simulink model "control_core"  (R2022b)
settings: Solver=FixedStepAuto  StartTime=0.0  StopTime=60  FixedStep=.01  RelTol=1e-3
undefined symbols (not defined in the file): airframe, CdProp, Cdx, Cdy, Cdz, Ct, Earth, g, Ixx, Iyy, Izz, Jr, larm, mass, WGS84
libraries: slpidlib x6, aerolibutil x3, vrlib x3, sharedtransform x2, shared6dof x2, simulink_extras x2, simulink x2, aerolibfltsims x1, aerolibtransform2 x1
(part 2 of 2)

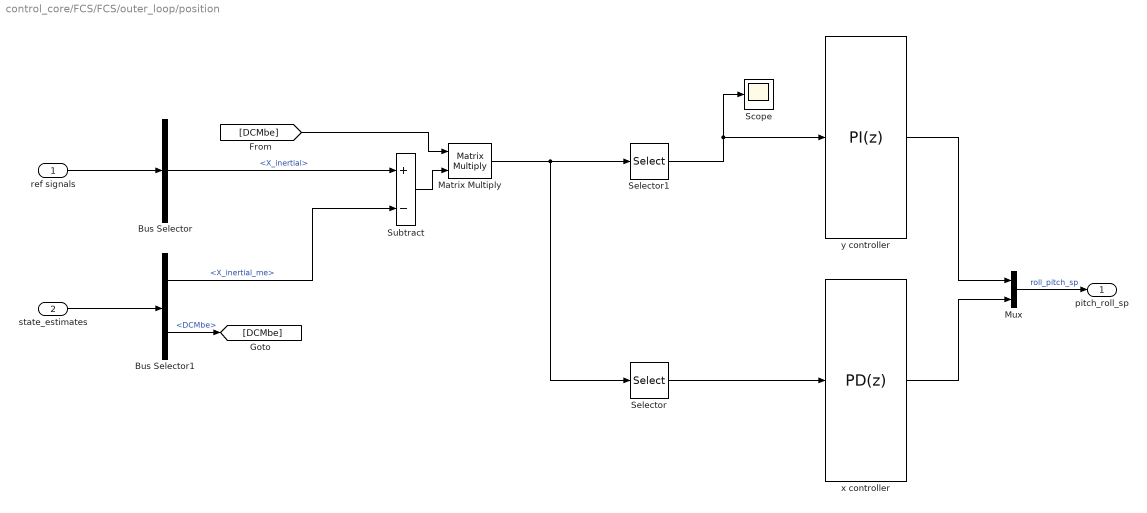
== system control_core/FCS/FCS/outer_loop/position ==
  ref signals : Inport
  state_estimates : Inport  Port=2
  Bus Selector : BusSelector  OutputSignals=X_inertial
  Bus Selector1 : BusSelector  OutputSignals=X_inertial_me,DCMbe
  Matrix Multiply : Product  Multiplication=Matrix(*)
  Mux : Mux  Inputs=2
  Scope : Scope
  Selector : Selector  InputPortWidth=3  IndexOptions=Index vector (dialog)  Indices=[1]  OutputSizes=1
  Selector1 : Selector  InputPortWidth=3  IndexOptions=Index vector (dialog)  Indices=[2]  OutputSizes=1
  Subtract : Sum  Inputs=+-
  x controller : slpidlib/PID Controller  Controller=PD  Form=Parallel  TimeDomain=Discrete-time  UseExternalTs=off  SampleTime=-1  IntegratorMethod=Forward Euler  FilterMethod=Forward Euler  ControllerParametersSource=internal  P=-0.0205622316535753  I=.000001  UseKiTs=off  D=0  N=100  UseFilter=on  TunerSelectOption=Transfer Function Based (PID Tuner App)  InitialConditionSource=internal  InitialConditionForIntegrator=0  InitialConditionForFilter=0  DifferentiatorICPrevScaledInput=0  ExternalReset=none  TrackingMode=off  Kt=1  LimitOutput=off  SatLimitsSource=internal  UpperSaturationLimit=inf  LowerSaturationLimit=-inf  LinearizeAsGain=on  AntiWindupMode=clamping  Kb=1  LimitIntegrator=off  UpperIntegratorSaturationLimit=inf  LowerIntegratorSaturationLimit=-inf  POutMin=[]  POutMax=[]  IOutMin=[]  IOutMax=[]  DOutMin=[]  DOutMax=[]  NOutMin=[]  NOutMax=[]  SumOutMin=[]  SumOutMax=[]  SaturationOutMin=[]  SaturationOutMax=[]  PParamMin=[]  PParamMax=[]  IParamMin=[]  IParamMax=[]  DParamMin=[]  DParamMax=[]  NParamMin=[]  NParamMax=[]  KbParamMin=[]  KbParamMax=[]  KtParamMin=[]  KtParamMax=[]  KbOutMin=[]  KbOutMax=[]  KtOutMin=[]  KtOutMax=[]  IntegratorOutMin=[]  IntegratorOutMax=[]  FilterOutMin=[]  FilterOutMax=[]  SumI1OutMin=[]  SumI1OutMax=[]  SumI2OutMin=[]  SumI2OutMax=[]  SumI3OutMin=[]  SumI3OutMax=[]  SumI4OutMin=[]  SumI4OutMax=[]  SumDOutMin=[]  SumDOutMax=[]  DifferentiatorOutMin=[]  DifferentiatorOutMax=[]  FilterDiffOutCoefMin=[]  FilterDiffOutCoefMax=[]  ReciprocalOutMin=[]  ReciprocalOutMax=[]  SumDenOutMin=[]  SumDenOutMax=[]  SumNumOutMin=[]  SumNumOutMax=[]  DivideOutMin=[]  DivideOutMax=[]  UdiffTsProdOutMin=[]  UdiffTsProdOutMax=[]  NTsProdOutMin=[]  NTsProdOutMax=[]  UintegralTsProdOutMin=[]  UintegralTsProdOutMax=[]  UngainTsProdOutMin=[]  UngainTsProdOutMax=[]  ClampingZeroOutDataTypeStr=Inherit: Inherit via back propagation  ClampingZeroOutMin=[]  ClampingZeroOutMax=[]  FilterDenConstantOutDataTypeStr=Inherit: Inherit via back propagation  FilterDenConstantOutMin=[]  FilterDenConstantOutMax=[]  PCopyOutDataTypeStr=Inherit: Inherit via back propagation  PCopyOutMin=[]  PCopyOutMax=[]  NCopyOutDataTypeStr=Inherit: Inherit via back propagation  NCopyOutMin=[]  NCopyOutMax=[]  IntegratorContinuousStateAttributes=''  IntegratorStateMustResolveToSignalObject=off  IntegratorRTWStateStorageClass=Auto  FilterContinuousStateAttributes=''  FilterStateMustResolveToSignalObject=off  FilterRTWStateStorageClass=Auto  ParallelPVariant=InternalParameters  IdealPVariant=Disabled  IVariant=Disabled  DVariant=InternalParameters  IntegratorVariant=Disabled  SatVariant=Disabled  AWVariant=Disabled  PCopyVariant=Disabled  TRVariant=Disabled  FdbkBlocksVariant=Forward  IdealPFdbkVariant=Disabled  SatFdbkVariant=Disabled  DerivativeFilterVariant=ForwardEulerFilter  NVariant=InternalParameters  NCopyVariant=Disabled  FilterICVariant=InternalICsFilter  IntegratorICVariant=Disabled  ExternalResetVariant=Disabled  TRSumVariant=Passthrough  SumFdbkVariant=Disabled  SumVariant=Sum_PD  TsampFilterVariant=InternalTs  TsampNgainVariant=Passthrough  TsampIntegralVariant=Disabled_SignalSpec  ExternalSaturationOutDataTypeStr=Inherit: Same as second input
  y controller : slpidlib/PID Controller  Controller=PI  Form=Parallel  TimeDomain=Discrete-time  UseExternalTs=off  SampleTime=-1  IntegratorMethod=Forward Euler  FilterMethod=Forward Euler  ControllerParametersSource=internal  P=0.0214287173644059  I=8.55230649524744e-05  UseKiTs=off  D=0  N=100  UseFilter=on  TunerSelectOption=Transfer Function Based (PID Tuner App)  InitialConditionSource=internal  InitialConditionForIntegrator=0  InitialConditionForFilter=0  DifferentiatorICPrevScaledInput=0  ExternalReset=none  TrackingMode=off  Kt=1  LimitOutput=off  SatLimitsSource=internal  UpperSaturationLimit=inf  LowerSaturationLimit=-inf  LinearizeAsGain=on  AntiWindupMode=clamping  Kb=1  LimitIntegrator=off  UpperIntegratorSaturationLimit=inf  LowerIntegratorSaturationLimit=-inf  POutMin=[]  POutMax=[]  IOutMin=[]  IOutMax=[]  DOutMin=[]  DOutMax=[]  NOutMin=[]  NOutMax=[]  SumOutMin=[]  SumOutMax=[]  SaturationOutMin=[]  SaturationOutMax=[]  PParamMin=[]  PParamMax=[]  IParamMin=[]  IParamMax=[]  DParamMin=[]  DParamMax=[]  NParamMin=[]  NParamMax=[]  KbParamMin=[]  KbParamMax=[]  KtParamMin=[]  KtParamMax=[]  KbOutMin=[]  KbOutMax=[]  KtOutMin=[]  KtOutMax=[]  IntegratorOutMin=[]  IntegratorOutMax=[]  FilterOutMin=[]  FilterOutMax=[]  SumI1OutMin=[]  SumI1OutMax=[]  SumI2OutMin=[]  SumI2OutMax=[]  SumI3OutMin=[]  SumI3OutMax=[]  SumI4OutMin=[]  SumI4OutMax=[]  SumDOutMin=[]  SumDOutMax=[]  DifferentiatorOutMin=[]  DifferentiatorOutMax=[]  FilterDiffOutCoefMin=[]  FilterDiffOutCoefMax=[]  ReciprocalOutMin=[]  ReciprocalOutMax=[]  SumDenOutMin=[]  SumDenOutMax=[]  SumNumOutMin=[]  SumNumOutMax=[]  DivideOutMin=[]  DivideOutMax=[]  UdiffTsProdOutMin=[]  UdiffTsProdOutMax=[]  NTsProdOutMin=[]  NTsProdOutMax=[]  UintegralTsProdOutMin=[]  UintegralTsProdOutMax=[]  UngainTsProdOutMin=[]  UngainTsProdOutMax=[]  ClampingZeroOutDataTypeStr=Inherit: Inherit via back propagation  ClampingZeroOutMin=[]  ClampingZeroOutMax=[]  FilterDenConstantOutDataTypeStr=Inherit: Inherit via back propagation  FilterDenConstantOutMin=[]  FilterDenConstantOutMax=[]  PCopyOutDataTypeStr=Inherit: Inherit via back propagation  PCopyOutMin=[]  PCopyOutMax=[]  NCopyOutDataTypeStr=Inherit: Inherit via back propagation  NCopyOutMin=[]  NCopyOutMax=[]  IntegratorContinuousStateAttributes=''  IntegratorStateMustResolveToSignalObject=off  IntegratorRTWStateStorageClass=Auto  FilterContinuousStateAttributes=''  FilterStateMustResolveToSignalObject=off  FilterRTWStateStorageClass=Auto  ParallelPVariant=InternalParameters  IdealPVariant=Disabled  IVariant=InternalParameters  DVariant=Disabled  IntegratorVariant=Discrete  SatVariant=Disabled  AWVariant=Passthrough  PCopyVariant=Disabled  TRVariant=Disabled  FdbkBlocksVariant=Forward  IdealPFdbkVariant=Disabled  SatFdbkVariant=Disabled  DerivativeFilterVariant=Disabled  NVariant=Disabled  NCopyVariant=Disabled_SignalSpec  FilterICVariant=Disabled  IntegratorICVariant=InternalICs  ExternalResetVariant=Disabled  TRSumVariant=Passthrough  SumFdbkVariant=Disabled  SumVariant=Sum_PI  TsampFilterVariant=InternalTs  TsampNgainVariant=Passthrough  TsampIntegralVariant=Passthrough  ExternalSaturationOutDataTypeStr=Inherit: Same as second input
  pitch_roll_sp : Outport
  wires:
  ref signals/1 -> Bus Selector/1
  state_estimates/1 -> Bus Selector1/1
  Bus Selector/1 -> Subtract/1  "<X_inertial>"
  Bus Selector1/1 -> Subtract/2  "<X_inertial_me>"
  Subtract/1 -> Matrix Multiply/2
  [DCMbe] -> Matrix Multiply/1
  Bus Selector1/2 -> [DCMbe]  "<DCMbe>"
  Matrix Multiply/1 -> Selector/1, Selector1/1
  Selector/1 -> x controller/1
  Selector1/1 -> y controller/1, Scope/1
  Mux/1 -> pitch_roll_sp/1  "roll_pitch_sp"
  x controller/1 -> Mux/2
  y controller/1 -> Mux/1

== system control_core/FCS/FCS/outer_loop/Altitude/Altitude PID ==
  altitude_setpoint : Inport
  altitude_feedback : Inport  Port=2
  Constant : Constant  Value=-g*mass
  PID Controller : slpidlib/PID Controller  Controller=PD  Form=Parallel  TimeDomain=Discrete-time  UseExternalTs=off  SampleTime=-1  IntegratorMethod=Forward Euler  FilterMethod=Forward Euler  ControllerParametersSource=internal  P=0.391711979722748  I=0  UseKiTs=off  D=0.101719151159153  N=0.643160901514191  UseFilter=on  TunerSelectOption=Transfer Function Based (PID Tuner App)  InitialConditionSource=internal  InitialConditionForIntegrator=0  InitialConditionForFilter=0  DifferentiatorICPrevScaledInput=0  ExternalReset=none  TrackingMode=off  Kt=1  LimitOutput=off  SatLimitsSource=internal  UpperSaturationLimit=inf  LowerSaturationLimit=-inf  LinearizeAsGain=on  AntiWindupMode=clamping  Kb=1  LimitIntegrator=off  UpperIntegratorSaturationLimit=inf  LowerIntegratorSaturationLimit=-inf  POutMin=[]  POutMax=[]  IOutMin=[]  IOutMax=[]  DOutMin=[]  DOutMax=[]  NOutMin=[]  NOutMax=[]  SumOutMin=[]  SumOutMax=[]  SaturationOutMin=[]  SaturationOutMax=[]  PParamMin=[]  PParamMax=[]  IParamMin=[]  IParamMax=[]  DParamMin=[]  DParamMax=[]  NParamMin=[]  NParamMax=[]  KbParamMin=[]  KbParamMax=[]  KtParamMin=[]  KtParamMax=[]  KbOutMin=[]  KbOutMax=[]  KtOutMin=[]  KtOutMax=[]  IntegratorOutMin=[]  IntegratorOutMax=[]  FilterOutMin=[]  FilterOutMax=[]  SumI1OutMin=[]  SumI1OutMax=[]  SumI2OutMin=[]  SumI2OutMax=[]  SumI3OutMin=[]  SumI3OutMax=[]  SumI4OutMin=[]  SumI4OutMax=[]  SumDOutMin=[]  SumDOutMax=[]  DifferentiatorOutMin=[]  DifferentiatorOutMax=[]  FilterDiffOutCoefMin=[]  FilterDiffOutCoefMax=[]  ReciprocalOutMin=[]  ReciprocalOutMax=[]  SumDenOutMin=[]  SumDenOutMax=[]  SumNumOutMin=[]  SumNumOutMax=[]  DivideOutMin=[]  DivideOutMax=[]  UdiffTsProdOutMin=[]  UdiffTsProdOutMax=[]  NTsProdOutMin=[]  NTsProdOutMax=[]  UintegralTsProdOutMin=[]  UintegralTsProdOutMax=[]  UngainTsProdOutMin=[]  UngainTsProdOutMax=[]  ClampingZeroOutDataTypeStr=Inherit: Inherit via back propagation  ClampingZeroOutMin=[]  ClampingZeroOutMax=[]  FilterDenConstantOutDataTypeStr=Inherit: Inherit via back propagation  FilterDenConstantOutMin=[]  FilterDenConstantOutMax=[]  PCopyOutDataTypeStr=Inherit: Inherit via back propagation  PCopyOutMin=[]  PCopyOutMax=[]  NCopyOutDataTypeStr=Inherit: Inherit via back propagation  NCopyOutMin=[]  NCopyOutMax=[]  IntegratorContinuousStateAttributes=''  IntegratorStateMustResolveToSignalObject=off  IntegratorRTWStateStorageClass=Auto  FilterContinuousStateAttributes=''  FilterStateMustResolveToSignalObject=off  FilterRTWStateStorageClass=Auto  ParallelPVariant=InternalParameters  IdealPVariant=Disabled  IVariant=Disabled  DVariant=InternalParameters  IntegratorVariant=Disabled  SatVariant=Disabled  AWVariant=Disabled  PCopyVariant=Disabled  TRVariant=Disabled  FdbkBlocksVariant=Forward  IdealPFdbkVariant=Disabled  SatFdbkVariant=Disabled  DerivativeFilterVariant=ForwardEulerFilter  NVariant=InternalParameters  NCopyVariant=Disabled  FilterICVariant=InternalICsFilter  IntegratorICVariant=Disabled  ExternalResetVariant=Disabled  TRSumVariant=Passthrough  SumFdbkVariant=Disabled  SumVariant=Sum_PD  TsampFilterVariant=InternalTs  TsampNgainVariant=Passthrough  TsampIntegralVariant=Disabled_SignalSpec  ExternalSaturationOutDataTypeStr=Inherit: Same as second input
  Sum : Sum  Inputs=|+-
  Sum1 : Sum  Inputs=|++
  Out1 : Outport
  wires:
  Sum/1 -> PID Controller/1
  PID Controller/1 -> Sum1/1
  Constant/1 -> Sum1/2
  altitude_feedback/1 -> Sum/2
  Sum1/1 -> Out1/1
  altitude_setpoint/1 -> Sum/1

== matlab function control_core/Quadcopter Dynamics, 'x'/MATLAB Function4 ==
  data: w_body input; d_euler output size=3; euler input
function d_euler = calc_euler_change(w_body, euler)

phi = euler(1);
theta = euler(2);
psi = euler(3);

p = w_body(1);
q = w_body(2);
r = w_body(3);

d_phi = p + (q*sin(phi) + r*cos(phi)) * tan(theta);
d_theta = q*cos(phi) - r*sin(phi);
d_psi = (q*sin(phi) + r*cos(phi))*(1/cos(theta));

d_euler = [d_phi; d_theta; d_psi];

== matlab function control_core/Quadcopter Dynamics, 'x'/MATLAB Function5 ==
  data: euler input; d_X output size=3; v_b input
function d_X = calc_inertial_velocity(euler, v_b)

phi = euler(1);
theta = euler(2);
psi = euler(3);

u = v_b(1);
v = v_b(2);
w = v_b(3);

dx = cos(theta)*cos(psi)*u + (-cos(phi)*sin(psi) + sin(phi)*sin(theta)*cos(psi))*v +...
    (sin(phi)*sin(psi)+cos(phi)*sin(theta)*cos(psi))*w;

dy = cos(theta)*sin(psi)*u + (cos(phi)*cos(psi)+sin(phi)*sin(theta)*sin(psi))*v + ...
    (-sin(phi)*cos(psi)+cos(phi)*sin(theta)*sin(psi))*w;

dz = (-sin(theta)*u+sin(phi)*cos(theta)*v+cos(phi)*cos(theta)*w);
d_X = [dx; dy; dz];

== matlab function control_core/FCS/Motor Mixing/MATLAB Function ==
  data: controlMatInv output; Ct parameter; larm parameter; CdProp parameter
function controlMatInv = calc_motor_speed(Ct,...
larm, CdProp)
% u1 = force;
% u2 = torques(1);
% u3 = torques(2);
% u4 = torques(3);


K = Ct;
L = larm;
C = CdProp;

% invControlMat = -[(C*u2 + C*u3 + C*L*u1 + K*L*u4)/(4*C*K*L);
%  (C*u2 - C*u3 - C*L*u1 + K*L*u4)/(4*C*K*L);
%  (C*u2 + C*u3 - C*L*u1 - K*L*u4)/(4*C*K*L);
% -(C*u2 - C*u3 + C*L*u1 - K*L*u4)/(4*C*K*L)];

invControlMat = [-1/(4*K), -1/(4*K*L), -1/(4*K*L), -1/(4*C);
                -1/(4*K),  1/(4*K*L), -1/(4*K*L),  1/(4*C);
                -1/(4*K),  1/(4*K*L),  1/(4*K*L), -1/(4*C);
                -1/(4*K), -1/(4*K*L),  1/(4*K*L),  1/(4*C)];
controlMatInv = invControlMat;

== matlab function control_core/Quadrotor Plant ('+')/p q r to DCM and Euler Angles/MATLAB Function ==
  data: wBody input; eulerAngleRates output; eulerAngles input
function eulerAngleRates = fcn(wBody,eulerAngles)

% Inertial frame angular velocities
phi = eulerAngles(1);
theta = eulerAngles(2);
psi = eulerAngles(3);
p = wBody(1);
q = wBody(2);
r = wBody(3);

rotMat = [1 sin(phi)*tan(theta) cos(phi)*tan(theta);
    0 cos(phi) -sin(phi);
    0 sin(phi)/cos(theta) cos(phi)/cos(theta)];
eulerAngleRates = rotMat*wBody;

% phidot = p+(q*sin(phi)+r*cos(phi))*tan(theta);
% thetadot = q*cos(phi)-r*sin(phi);
% psidot = (q*sin(phi)+r*cos(phi))/cos(theta);


% eulerAngleRates = [phidot;thetadot;psidot];


% rotBodytoInertial = [1 sin(phi)*sin(theta)/cos(theta) cos(phi)*sin(theta)/cos(theta);
%     0 cos(phi) -sin(phi);
%     0 sin(phi)/cos(theta) cos(phi)/cos(theta)];
% 
% eulerAngleRates = rotBodytoInertial*wBody;

== matlab function control_core/MATLAB Function2 ==
  data: w_actuator input; T output size=3; Moment output size=3; Ct parameter; larm parameter; CdProp parameter
function [T, Moment] = calc_actuator_force_moment(w_actuator, Ct, larm, CdProp)

K = Ct;
L_arm = larm;
C = CdProp;


w1 = w_actuator(1)^2;
w2 = w_actuator(2)^2;
w3 = w_actuator(3)^2;
w4 = w_actuator(4)^2;

T = [0; 0; -K * (sum(w_actuator.^2))];
L = K*L_arm*(-w1 + w2 + w3 - w4);
M = K*L_arm*(-w1 - w2 + w3 + w4);
N = C*(-w1 - w3 + w2 + w4);

Moment = [L; M; N];

== matlab function control_core/Quadrotor Plant ('+')/p q r to DCM and Euler Angles/MATLAB Function1 ==
  data: eulerAngles input; DCM output
function DCM = fcn(eulerAngles)

phi = eulerAngles(1);
theta = eulerAngles(2);
psi = eulerAngles(3);


DCM = [cos(psi)*cos(phi)-cos(theta)*sin(phi)*sin(psi), cos(psi)*sin(phi)+cos(theta)*cos(phi)*sin(psi), sin(psi)*sin(theta);
    -sin(psi)*cos(phi)-cos(theta)*sin(phi)*cos(psi) -sin(psi)*sin(phi)+cos(theta)*cos(phi)*cos(psi) cos(psi)*sin(theta);
    sin(theta)*sin(phi) -sin(theta)*cos(phi) cos(theta)];

== matlab function control_core/Quadrotor Plant ('+')/MATLAB Function4 ==
  data: DCM output; phi input; theta input; psi input
function DCM = DCM_body_to_inertial(phi,theta,psi)

% Performs a ZYX roation to rotate from body to inertial coordinate frame
% 
DCM = [cos(theta)*cos(psi), cos(theta)*sin(psi), -sin(theta);...
    -sin(psi)*cos(phi)+sin(theta)*sin(phi)*cos(psi), cos(psi)*cos(phi)+sin(phi)*sin(theta)*sin(psi), sin(phi)*cos(theta);...
    sin(phi)*sin(psi)+cos(phi)*sin(theta)*cos(psi), -sin(phi)*cos(psi)+cos(phi)*sin(theta)*sin(psi), cos(theta)*cos(phi)];
    

DCM = DCM';

% % % Trans_mat1=[(cos(psi)*cos(theta)), (-sin(psi)*cos(phi)+cos(psi)*sin(theta)*sin(phi)), (sin(psi)*sin(phi)+cos(psi)*sin(theta)*cos(phi));...
% % %           (sin(psi)*cos(theta)), (cos(psi)*cos(phi)+sin(theta)*sin(psi)*sin(phi)), (-cos(psi)*sin(phi)+sin(theta)*sin(psi)*cos(phi));...
% % %           (-sin(theta)), (cos(theta)*sin(phi)), (cos(theta)*cos(phi))];
% % %       
% % % 
% % % 
% % % R_phi=[1, 0, 0;...
% % %        0, cos(phi), sin(phi);...
% % %        0, -sin(phi), cos(phi)];
% % %    
% % % R_theta=[cos(theta), 0, -sin(theta);...
% % %         0, 1, 0;...
% % %         sin(theta), 0, cos(theta)];
% % % 
% % % R_psi=[cos(psi), sin(psi), 0;...
% % %        -sin(psi), cos(psi), 0;...
% % %        0, 0, 1];
% % %    
% % %   Trans_mat= R_psi*R_theta*R_phi;
% % %   DCM=Trans_mat;

== matlab function control_core/Quadrotor Plant ('+')/MATLAB Function5 ==
  data: omegaMotor input; wPhi_dot output; Torques input; JMatrix input; wBody input; JrProp input; wTheta_dot output; wPsi_dot output
function [wPhi_dot,wTheta_dot,wPsi_dot] = fcn(omegaMotor,Torques,JMatrix,wBody,JrProp)

Ixx = JMatrix(1,1);
Iyy = JMatrix(2,2);
Izz = JMatrix(3,3);

wPhi = wBody(1);
wTheta = wBody(2);
wPsi = wBody(3);

omegaR = omegaMotor(1)-omegaMotor(2)+omegaMotor(3)-omegaMotor(4);

wPhi_dot = ((Iyy-Izz)*wTheta*wPsi+JrProp*omegaR*wTheta+Torques(1))/Ixx;
wTheta_dot = ((Izz-Ixx)*wPhi*wPsi-JrProp*omegaR*wPhi+Torques(2))/Iyy;
wPsi_dot = ((Ixx-Iyy)*wTheta*wPhi+Torques(3))/Izz;

== matlab function control_core/Quadcopter Dynamics, 'x'/MATLAB Function ==
  data: euler input; dv_body output size=3; w_b input; v_b input; g parameter
function dv_body = calc_body_vel_change(euler, w_b, v_b, g)

u = v_b(1);
v = v_b(2);
w = v_b(3);

theta = euler(2);
phi = euler(1);
psi = euler(3);

p = w_b(1);
q = w_b(2);
r = w_b(3);


du = -g*sin(theta)+r*v - q*w;
dv = g*sin(phi)*cos(theta) - r*u + p*w;
dw = g*cos(phi)*cos(theta) + q*u - p*v;

dv_body = [du; dv; dw];

== matlab function control_core/Quadcopter Dynamics, 'x'/MATLAB Function2 ==
  data: v_inertial input; drag output size=3; Cdx parameter; Cdy parameter; Cdz parameter; mass parameter
function drag = calc_drag(v_inertial, Cdx, Cdy, Cdz, mass)

dx = v_inertial(1);
dy = v_inertial(2);
dz = v_inertial(3);

Fd_x = -(1/mass)*Cdx*dx;
Fd_y = -(1/mass)*Cdy*dy;
Fd_z = -(1/mass)*Cdz*dz;

drag = [Fd_x; Fd_y; Fd_z];

== matlab function control_core/Quadcopter Dynamics, 'x'/MATLAB Function3 ==
  data: w_b input; dw_body output single size=3; w_prop input single; Moments input single; Ixx parameter; Iyy parameter; Izz parameter; Jr parameter
function dw_body = calc_body_rate_change(w_b, w_prop, Moments, ...
Ixx, Iyy, Izz, Jr)

L = Moments(1);
M = Moments(2);
N = Moments(3);

omega_p = -w_prop(1) + w_prop(2) - w_prop(3) + w_prop(4);


p = w_b(1);
q = w_b(2);
r = w_b(3);

dp = (1/Ixx)*(L + (Iyy - Izz)*q*r) + q*omega_p*Jr/Ixx;
dq = (1/Iyy)*(M + (Izz - Ixx)*p*r) - p*omega_p*Jr/Iyy;
% dp = (1/Ixx)*(L + (Iyy - Izz)*q*r);
% dq = (1/Iyy)*(M + (Izz - Ixx)*p*r);
dr = (1/Izz)*(N + (Ixx - Iyy)*p*q);

dw_body = [dp; dq; dr];
